simulink model "boostObserver_old"  (R2020a)
settings: Solver=VariableStepAuto  StartTime=0.0  StopTime=3.2  FixedStep=0.0005  MaxStep=9e-06  RelTol=1e-03  EnableMultiTasking=on
InitFcn:
  | kp=0.01;
  | ki=0.01;
  | 
  | k=2;
  | em=100000000;
  | GE=1/em;
  | GU=k*ki/GE;
  | GCE=k*kp/GU;
model workspace (MAT data in the model file):
  time = 0.8
values from neighbouring files (symbols this model uses):
  A1 = obj.boostConverter.A1    [BoostController.m]    (also in BoostConverter.m = [-obj.R/obj.L 0;0 -1/(obj.Ro*obj.C)]; BuckBoostConverter.m = [-obj.R/obj.L 0;0 -1/(obj.Ro*obj.C)]; obsmc.m = Asigma{1,1}; workspace_atual.mat = [-16.4  0; 0  -3.50877192982])
  A2 = obj.boostConverter.A2    [BoostController.m]    (also in BoostConverter.m = [-obj.R/obj.L -1/obj.L;1/obj.C -1/(obj.Ro*obj.C)]; BuckBoostConverter.m = [-obj.R/obj.L 1/obj.L;-1/obj.C -1/(obj.Ro*obj.C)]; obsmc.m = Asigma{1,2}; workspace_atual.mat = [-16.4  -200; 350.877192982  -3.50877192982])
  AlarmDeadTime = 0.50    (= 0.5)    [BoostFaultSimulation.m]    (also in workspace_atual.mat; workspace_certo.mat)
  B1 = obj.boostConverter.B1    [BoostController.m]    (also in BoostConverter.m = [1/obj.L;0]; BuckBoostConverter.m = [1/obj.L;0]; obsmc.m = Bsigma{1,1}; workspace_atual.mat = [200 0])
  boost_parameters = [obj.Ro,obj.R,obj.L,obj.C,obj.u]'    [BoostConverter.m]    (also in BuckBoostConverter.m; boostResults2Latex.m = boost.parameters(); workspace_atual.mat = [100 0.082 0.005 0.00285 190]; workspace_certo.mat = [100 0.082 0.005 0.00285 190])
  C = 1e-3    (= 0.001)    [boostResults2Latex.m]
  CiL = [0 1]    [workspace_atual.mat]    (also in workspace_certo.mat)
  Cmatrix = [1  0; 0  1]    [workspace_atual.mat]    (also in workspace_certo.mat)
  CVc = [1 0]    [workspace_atual.mat]    (also in workspace_certo.mat)
  D1 = [1  0; 0  1]    [workspace_atual.mat]    (also in workspace_certo.mat)
  FaultClass = 0    [BoostFaultSimulation.m]    (also in workspace_atual.mat = 1; workspace_certo.mat = 1)
  iLFaultSwitch = 0    [BoostFaultSimulation.m]    (also in workspace_atual.mat; workspace_certo.mat)
  iLFaultTime = 1.70    (= 1.7)    [BoostFaultSimulation.m]    (also in workspace_atual.mat; workspace_certo.mat)
  iLGainFaultFactor = 15    [BoostFaultSimulation.m]    (also in workspace_atual.mat; workspace_certo.mat)
  iLNoiseFaultSwitch = 0    [BoostFaultSimulation.m]    (also in workspace_atual.mat; workspace_certo.mat)
  iLNoiseTime = 1.70    (= 1.7)    [BoostFaultSimulation.m]    (also in workspace_atual.mat; workspace_certo.mat)
  Jth = 2000    [workspace_atual.mat]    (also in workspace_certo.mat)
  L = 1e-3    (= 0.001)    [boostResults2Latex.m]    (also in obsmc.m = sdpvar(3,1,'full'))
  LoadAddResistor = obj.LoadAddFactor*obj.Ro    [BoostFaultSimulation.m]    (also in workspace_atual.mat = 30; workspace_certo.mat = 30)
  LoadAddSignalSwitch = 1    [BoostFaultSimulation.m]    (also in workspace_atual.mat; workspace_certo.mat)
  LoadAddSwitch = 0    [BoostFaultSimulation.m]    (also in workspace_atual.mat; workspace_certo.mat)
  LoadAddTime = 0.90    (= 0.9)    [BoostFaultSimulation.m]    (also in workspace_atual.mat; workspace_certo.mat)
  LoadRemoveResistor = obj.Ro*(1-obj.LoadRemoveFactor)/(obj.LoadRemoveFactor)    [BoostFaultSimulation.m]    (also in workspace_atual.mat = 233.333333333; workspace_certo.mat = 233.333333333)
  LoadRemoveSignalSwitch = 1    [BoostFaultSimulation.m]    (also in workspace_atual.mat; workspace_certo.mat)
  LoadRemoveSwitch = 0    [BoostFaultSimulation.m]    (also in workspace_atual.mat; workspace_certo.mat)
  LoadRemoveTime = 0.90    (= 0.9)    [BoostFaultSimulation.m]    (also in workspace_atual.mat; workspace_certo.mat)
  LobsiL = [1737913.15707 66180.0912281]    [workspace_atual.mat]    (also in workspace_certo.mat)
  LobsVc = [61200 1]    [workspace_atual.mat]    (also in workspace_certo.mat)
  ObsEp = 70    [workspace_atual.mat]    (also in workspace_certo.mat)
  R = 0.1    [boostResults2Latex.m]    (also in workspace_atual.mat = 0.082; workspace_certo.mat = 0.082)
  ReconfigDelay = 0    [BoostFaultSimulation.m]    (also in workspace_atual.mat = 0.2; workspace_certo.mat = 0.2)
  ReconfigSwitch = 0    [BoostFaultSimulation.m]    (also in workspace_atual.mat; workspace_certo.mat)
  ReconfigTime = 1.707    [BoostFaultSimulation.m]    (also in workspace_atual.mat; workspace_certo.mat)
  rho = 5    [workspace_atual.mat]    (also in workspace_certo.mat)
  RMSfrequency = 47.61    [BoostFaultSimulation.m]    (also in workspace_atual.mat; workspace_certo.mat)
  Ro = 100    [BoostFaultSimulation.m]    (also in boostResults2Latex.m = 10; workspace_atual.mat; workspace_certo.mat)
  Smep = 80    [workspace_atual.mat]    (also in workspace_certo.mat)
  SourceAddSignalSwitch = 1    [BoostFaultSimulation.m]    (also in workspace_atual.mat; workspace_certo.mat)
  SourceAddSwitch = 0    [BoostFaultSimulation.m]    (also in workspace_atual.mat; workspace_certo.mat)
  SourceAddTime = 0.90    (= 0.9)    [BoostFaultSimulation.m]    (also in workspace_atual.mat; workspace_certo.mat)
  SourceAddVoltage = obj.SourceAddFactor*obj.u    [BoostFaultSimulation.m]    (also in workspace_atual.mat = 19; workspace_certo.mat = 19)
  SourceRemoveSignalSwitch = 1    [BoostFaultSimulation.m]    (also in workspace_atual.mat; workspace_certo.mat)
  SourceRemoveSwitch = 0    [BoostFaultSimulation.m]    (also in workspace_atual.mat; workspace_certo.mat)
  SourceRemoveTime = 0.90    (= 0.9)    [BoostFaultSimulation.m]    (also in workspace_atual.mat; workspace_certo.mat)
  SourceRemoveVoltage = obj.SourceRemoveFactor*obj.u    [BoostFaultSimulation.m]    (also in workspace_atual.mat = 19; workspace_certo.mat = 19)
  ueq = 0.5    [workspace_atual.mat]    (also in workspace_certo.mat)
  VcFaultSwitch = 0    [BoostFaultSimulation.m]    (also in workspace_atual.mat; workspace_certo.mat)
  VcFaultTime = 1.70    (= 1.7)    [BoostFaultSimulation.m]    (also in workspace_atual.mat; workspace_certo.mat)
  VcGainFaultFactor = 15    [BoostFaultSimulation.m]    (also in workspace_atual.mat; workspace_certo.mat)
  VcNoiseFaultSwitch = 0    [BoostFaultSimulation.m]    (also in workspace_atual.mat; workspace_certo.mat)
  VcNoiseTime = 1.70    (= 1.7)    [BoostFaultSimulation.m]    (also in workspace_atual.mat; workspace_certo.mat)
  ve = 380    [BoostFaultSimulation.m]    (also in boostResults2Latex.m = 100; workspace_atual.mat; workspace_certo.mat)
  x_e = [ie;ve]    [BoostConverter.m]    (also in BuckBoostConverter.m)
  xe = obj.boostConverter.equilibriumstate(ve)    [BoostController.m]    (also in workspace_atual.mat = [7.62509288104 380]; workspace_certo.mat = [7.62509288104 380])
undefined symbols (not defined in the file or in its folder): Atilde1, Atilde2, Ctilde1, Dtilde1, Dtilde2, F, G, MAXnet, MINnet
libraries: neural x74, powerlib x70, dspstat3 x16, simulink x9, powerlib_meascontrol x7, dspmtrx3 x7, dspmathops x3
(part 2 of 7)

== system boostObserver_old/Subsystem/Fault Identification Neural Netowrk ==
  netInputs : Inport
  Constant : Constant  Commented=on  Value=MAXnet
  Constant1 : Constant  Commented=on  Value=[0;0;0]
  Constant4 : Constant  Commented=on  Value=MINnet
  Demux : Demux  Commented=on  Outputs=3
  Demux1 : Demux  Commented=on  Outputs=3
  Demux2 : Demux  Commented=on  Outputs=3
  Maximum : dspstat3/Maximum  operation=maximum  fcn=Value and Index  indexBase=One  operateOver=Each column  Dimension=1  InputProcessing=Columns as channels (frame based)  reset=None  roiEnable=off  roiType=Rectangles  roiPortion=Entire ROI  roiOutput=Individual statistics for each ROI  roiFlag=off  roundingMode=Floor  overflowMode=off  accumDataTypeStr=Inherit: Same as product output  accumLastDataTypeStr=Inherit: Same as product output
  Median Filter : dspstat3/Median Filter  Commented=on  WindowLength=1  SimulateUsing=Code generation
      settings: SourceProductBaseCode=DS
  Mux : Mux  Commented=on  Inputs=3
  Pattern Recognition Neural Network1 : Subsystem
      mask help: Pattern Recognition Neural Network
      mask Display: e = 0.06;c1 = [120 150 230]/255;c2 = ([120 150 230]+0)/383;c3 = ([120 150 230]+128)/383;patch([0 1 1 0],[0 0 1 1],c1);patch([0 1 1 1-e 1-e 0+e],[0 0 1 1-e 0+e 0+e],c2);patch([0 0 1 1-e 0+e 0+e],[0 1 1 1-e 1-e 0+e],c3);plot([0 1 1 0 0],[0 0 1 1 0]);fprintf('NNET');port_label('input',1,' Input');port_label('output',1,'Output ');
  Scope : Scope
  Scope1 : Scope
  Subsystem : Subsystem  Commented=on
  Subsystem1 : Subsystem  Commented=on
  Subsystem2 : Subsystem  Commented=on
  Terminator : Terminator
  netOutputs : Outport
  wires:
  Maximum/1 -> Terminator/1
  Maximum/2 -> Scope1/1, netOutputs/1, Scope/1
  Constant/1 -> Demux/1
  Demux2/1 -> Subsystem/1(input)
  Demux1/1 -> Subsystem/2(min)
  Demux/1 -> Subsystem/3(max)
  Demux1/2 -> Subsystem1/2(min)
  Demux/2 -> Subsystem1/3(max)
  Demux2/2 -> Subsystem1/1(input)
  Demux/3 -> Subsystem2/3(max)
  Demux1/3 -> Subsystem2/2(min)
  Demux2/3 -> Subsystem2/1(input)
  Subsystem/1(Out1) -> Mux/1
  Subsystem1/1(Out1) -> Mux/2
  Subsystem2/1(Out1) -> Mux/3
  Constant4/1 -> Demux1/1
  netInputs/1 -> Pattern Recognition Neural Network1/1(Input)
  Pattern Recognition Neural Network1/1(Output) -> Maximum/1

== system boostObserver_old/Subsystem/If Action Subsystem ==
  In1 : Inport
  Action Port : ActionPort  ActionPortLabel=case [ 1 6 ]:
  Out1 : Outport
  wires:
  In1/1 -> Out1/1

== system boostObserver_old/Subsystem/If Action Subsystem1 ==
  In1 : Inport
  Action Port : ActionPort  ActionPortLabel=default:
  Out1 : Outport
  wires:
  In1/1 -> Out1/1

== system boostObserver_old/Subsystem/If Action Subsystem2 ==
  y : Inport
  Action Port : ActionPort  ActionPortLabel=case [ 4 5 ]:
  x_hat : Outport
  wires:
  y/1 -> x_hat/1

== system boostObserver_old/Subsystem/If Action Subsystem4 ==
  y : Inport
  Action Port : ActionPort  ActionPortLabel=case [ 2 3 ]:
  x_hat : Outport
  wires:
  y/1 -> x_hat/1

== system boostObserver_old/Subsystem/Residual Generator2 ==
  e_y : Inport
  Matrix Square1 : dspmtrx3/Matrix Square  OutMin=[]  OutMax=[]
      settings: SourceProductBaseCode=DS
  Moving RMS : dspstat3/Moving RMS  Method=Sliding window  ForgettingFactorPort=off  SpecifyWindowLength=on  WindowLength=RMSfrequency/10  ForgettingFactor=0.9  SimulateUsing=Code generation
      settings: SourceProductBaseCode=DS
  Sqrt2 : Sqrt  SaturateOnIntegerOverflow=on
  RMS : Outport
  wires:
  Matrix Square1/1 -> Sqrt2/1
  e_y/1 -> Matrix Square1/1
  Sqrt2/1 -> Moving RMS/1
  Moving RMS/1 -> RMS/1

== system boostObserver_old/Subsystem/Sliding Mode Observer 5 ==
  ey : Inport
  v : Inport  Port=2
  sigma : Inport  Port=3
  C : Constant  Value=Ctilde1
  ObserverDynamics : Subsystem
  Product : Product  Multiplication=Matrix(*)
  ey_out : Outport
  y_e_tilde_hat : Outport  Port=2
  wires:
  Product/1 -> y_e_tilde_hat/1
  C/1 -> Product/1
  ObserverDynamics/1(e_tilde_hat) -> Product/2
  sigma/1 -> ObserverDynamics/3(sigma)
  ey/1 -> ey_out/1, ObserverDynamics/1(ey)
  v/1 -> ObserverDynamics/2(v)

== system boostObserver_old/Subsystem/Subsystem ==
  y : Inport
  C : Inport  Port=2
  y_hat : Inport  Port=3
  "    1" : Constant  Value=ObsEp
  Product : Product  Multiplication=Matrix(*)
  SlidingSurface : Subsystem
  Subtract : Sum  Inputs=+-
  error : Outport
  wires:
  Subtract/1 -> SlidingSurface/1(S)  "y-y_hat"
  Product/1 -> Subtract/1
  "    1"/1 -> SlidingSurface/2(ep)
  SlidingSurface/1(d) -> error/1
  y_hat/1 -> Subtract/2
  C/1 -> Product/1
  y/1 -> Product/2

== system boostObserver_old/Subsystem/Subsystem1 ==
  y : Inport
  C : Inport  Port=2
  y_hat : Inport  Port=3
  "    1" : Constant  Value=ObsEp
  Product : Product  Multiplication=Matrix(*)
  SlidingSurface : Subsystem
  Subtract : Sum  Inputs=+-
  error : Outport
  wires:
  Subtract/1 -> SlidingSurface/1(S)  "y-y_hat"
  Product/1 -> Subtract/1
  "    1"/1 -> SlidingSurface/2(ep)
  SlidingSurface/1(d) -> error/1
  y_hat/1 -> Subtract/2
  C/1 -> Product/1
  y/1 -> Product/2

== system boostObserver_old/Subsystem/Subsystem2 ==
  x : Inport
  xe : Inport  Port=2
  y_fault : Inport  Port=3
  Constant : Constant  Value=D1
  Matrix Multiply : Product  Multiplication=Matrix(*)
  Sum : Sum  Inputs=|++
  Sum1 : Sum  Inputs=|-+
  y_e : Gain  Gain=Cmatrix  Multiplication=Matrix(K*u)
  f_s : Outport
  wires:
  Matrix Multiply/1 -> f_s/1
  Constant/1 -> Matrix Multiply/1  "D^- = D"
  x/1 -> Sum/1
  xe/1 -> Sum/2
  Sum/1 -> y_e/1
  y_e/1 -> Sum1/2
  Sum1/1 -> Matrix Multiply/2
  y_fault/1 -> Sum1/1

== system boostObserver_old/Subsystem/Subsystem9 ==
  x : Inport
  Demux : Demux  Outputs=2
  Residual Generator2 : Subsystem
  VcRMS : Outport
  wires:
  x/1 -> Demux/1
  Demux/2 -> Residual Generator2/1(e_y)
  Residual Generator2/1(RMS) -> VcRMS/1

== system boostObserver_old/Subsystem/Vc OBserver ==
  ObserverError : Inport
  C : Inport  Port=2
  sigma : Inport  Port=3
  Constant : Constant  Value=LobsVc
  Product2 : Product  Multiplication=Matrix(*)
  calc_x_hat : Subsystem
  x_hat : Outport
  y_hat : Outport  Port=2
  wires:
  sigma/1 -> calc_x_hat/1(sigma)
  calc_x_hat/1(x_hat) -> Product2/2, x_hat/1
  Product2/1 -> y_hat/1
  C/1 -> Product2/1
  ObserverError/1 -> calc_x_hat/2(rsign)
  Constant/1 -> calc_x_hat/3(Lobs)

== system boostObserver_old/Subsystem/iL Observer ==
  C : Inport
  ObserverError : Inport  Port=2
  sigma : Inport  Port=3
  Constant8 : Constant  Value=LobsiL
  Product2 : Product  Multiplication=Matrix(*)
  calc_x_hat : Subsystem
  x_hat : Outport
  y_hat : Outport  Port=2
  wires:
  sigma/1 -> calc_x_hat/1(sigma)
  calc_x_hat/1(x_hat) -> Product2/2, x_hat/1
  Product2/1 -> y_hat/1
  C/1 -> Product2/1
  ObserverError/1 -> calc_x_hat/2(rsign)
  Constant8/1 -> calc_x_hat/3(Lobs)

== system boostObserver_old/Subsystem3/AntiFalseAlarm ==
  PRNN : Inport
  Alarm : Inport  Port=2
  Constant7 : Constant
  FaultDetecition1 : Switch  Criteria=u2 > Threshold
  Product1 : Product
  Step1 : Step  Time=AlarmDeadTime  SampleTime=0
  FaultClass : Outport
  AlarmOut : Outport  Port=2
  wires:
  PRNN/1 -> FaultDetecition1/1
  Constant7/1 -> FaultDetecition1/3
  Step1/1 -> Product1/1
  Alarm/1 -> Product1/2
  Product1/1 -> AlarmOut/1, FaultDetecition1/2
  FaultDetecition1/1 -> FaultClass/1

== system boostObserver_old/Subsystem3/Augmented Error Generator ==
  e : Inport
  Mux : Mux  Inputs=2
  z1 : Subsystem
  e_tilde : Outport
  wires:
  z1/1(z) -> Mux/2
  Mux/1 -> e_tilde/1
  e/1 -> Mux/1, z1/1(z_dot)

== system boostObserver_old/Subsystem3/Boost Converter ==
  note: Escolha do tipo de entrada
  note: Circuito do conversor
  sigma : Inport
  ConversorBoost : Subsystem
  Mux1 : Mux  Inputs=2
  Terminator : Terminator
  Terminator1 : Terminator
  TipoEntrada : Subsystem
  x : Outport
  wires:
  TipoEntrada/4("Rvariavel ") -> [Rinput]
  sigma/1 -> ConversorBoost/1(sigma)
  [Vinput1] -> ConversorBoost/2(Vinput1)
  [Vinput2] -> ConversorBoost/3(Vinput2)
  [Rinput] -> ConversorBoost/5(Rinput)
  TipoEntrada/5("Rparallelvariavel ") -> [Rparallelinput]
  [Rparallelinput] -> ConversorBoost/6(Rparallelinput)
  [Vinput3] -> ConversorBoost/4(Vinput3)
  TipoEntrada/1(Vu) -> [Vinput1]
  TipoEntrada/2(VuAdd) -> [Vinput2]
  TipoEntrada/3(VuRemove) -> [Vinput3]
  ConversorBoost/1(iLoutput) -> Mux1/1
  ConversorBoost/2(Vcoutput) -> Mux1/2
  Mux1/1 -> x/1
  ConversorBoost/3(iro) -> Terminator/1
  ConversorBoost/4(Vu) -> Terminator1/1

== system boostObserver_old/Subsystem3/Controlador1 ==
  note: Sinal de controle
  note: Superfície
  note: Ponto de equilíbrio
  ve : Inport
  x : Inport  Port=2
  "    " : Constant  Value=ueq
  "    2" : Constant  Value=Smep
  Constant6 : Constant  Value=boost_parameters
  Demux1 : Demux  Outputs=2
  Demux2 : Demux  Outputs=2
  Gain : Gain  Gain=0.8
  Gain1 : Gain  Gain=8
  Gain3 : Gain  Gain=2.3
  Integrator1 : Integrator
  PWM : powerlib_meascontrol/Pulse & Signal Generators/PWM Generator (DC-DC)  Fsw=7000  Ts=0
  SlidingSurface : Subsystem
  Sum : Sum  Inputs=|++
  Sum4 : Sum  Inputs=++|
  Sum5 : Sum  Inputs=-+|
  Sum6 : Sum  Inputs=-+|
  Sum9 : Sum  Inputs=|++
  xe : MATLAB Function  TreatAsAtomicUnit=on
  sigma : Outport
  i_e : Outport  Port=2
  x_e : Outport  Port=3
  wires:
  Demux1/1 -> Sum6/2  "IL"
  PWM/1 -> sigma/1
  ve/1 -> xe/2(ve)
  Demux2/2 -> Sum5/1  "Vo1"
  "    "/1 -> Sum9/2
  Sum6/1 -> Gain1/1
  Sum5/1 -> Gain3/1, Gain/1
  Sum9/1 -> PWM/1
  Demux1/2 -> Sum5/2  "Vo1"
  Demux2/1 -> Sum6/1
  xe/2(i_e) -> i_e/1
  x/1 -> Demux2/1
  Constant6/1 -> xe/1(boost_parameters)
  Gain1/1 -> Sum4/2
  xe/1(x_e) -> Demux1/1, x_e/1
  Gain/1 -> Sum/1
  Gain3/1 -> Integrator1/1
  Sum/1 -> Sum4/1
  SlidingSurface/1(d) -> Sum9/1
  "    2"/1 -> SlidingSurface/2(ep)
  Sum4/1 -> SlidingSurface/1(S)
  Integrator1/1 -> Sum/2

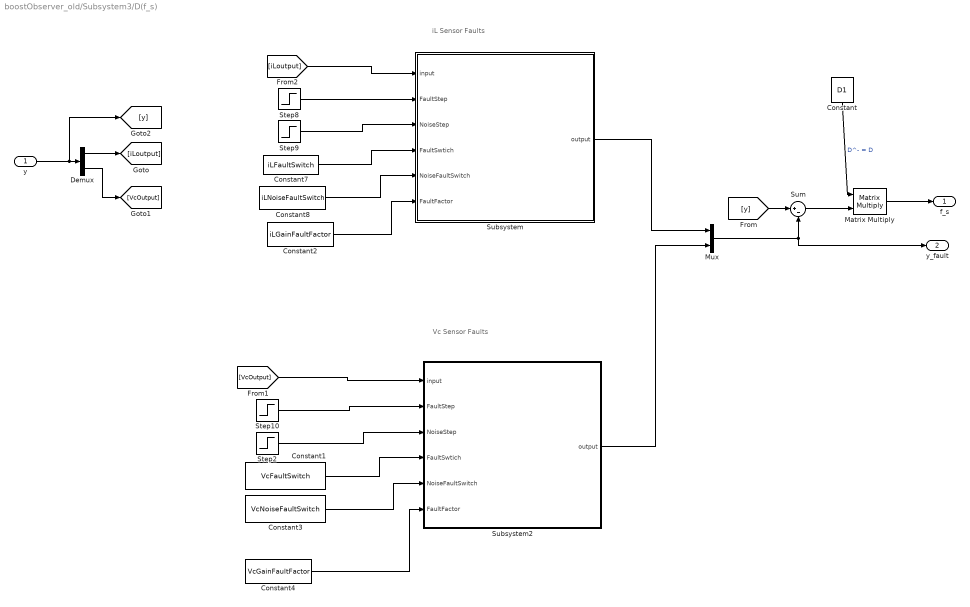
== system boostObserver_old/Subsystem3/D(f_s) ==
  note: iL Sensor Faults
  note: Vc Sensor Faults
  y : Inport
  Constant : Constant  Value=D1
  Constant1 : Constant  Value=VcFaultSwitch
  Constant2 : Constant  Value=iLGainFaultFactor
  Constant3 : Constant  Value=VcNoiseFaultSwitch
  Constant4 : Constant  Value=VcGainFaultFactor
  Constant7 : Constant  Value=iLFaultSwitch
  Constant8 : Constant  Value=iLNoiseFaultSwitch
  Demux : Demux  Outputs=2
  Matrix Multiply : Product  Multiplication=Matrix(*)
  Mux : Mux  Inputs=2
  Step10 : Step  Time=VcFaultTime  SampleTime=0
  Step2 : Step  Time=VcNoiseTime  SampleTime=0
  Step8 : Step  Time=iLFaultTime  SampleTime=0
  Step9 : Step  Time=iLNoiseTime  SampleTime=0
  Subsystem : Subsystem
  Subsystem2 : Subsystem
  Sum : Sum  Inputs=|+-
  f_s : Outport
  y_fault : Outport  Port=2
  wires:
  [iLoutput] -> Subsystem/1(input)
  Constant7/1 -> Subsystem/4(FaultSwtich)
  Constant8/1 -> Subsystem/5(NoiseFaultSwitch)
  Step8/1 -> Subsystem/2(FaultStep)
  Step9/1 -> Subsystem/3(NoiseStep)
  Constant1/1 -> Subsystem2/4(FaultSwtich)
  Constant3/1 -> Subsystem2/5(NoiseFaultSwitch)
  Step10/1 -> Subsystem2/2(FaultStep)
  Step2/1 -> Subsystem2/3(NoiseStep)
  Constant2/1 -> Subsystem/6(FaultFactor)
  Constant4/1 -> Subsystem2/6(FaultFactor)
  [VcOutput] -> Subsystem2/1(input)
  Demux/1 -> [iLoutput]
  Demux/2 -> [VcOutput]
  y/1 -> [y], Demux/1
  Subsystem/1(output) -> Mux/1
  Subsystem2/1(output) -> Mux/2
  Mux/1 -> Sum/2, y_fault/1
  [y] -> Sum/1
  Constant/1 -> Matrix Multiply/1  "D^- = D"
  Sum/1 -> Matrix Multiply/2
  Matrix Multiply/1 -> f_s/1

== system boostObserver_old/Subsystem3/ErrorGenerator ==
  y_e_tilde : Inport
  y_e_tilde_hat : Inport  Port=2
  AND : Logic  IconShape=distinctive  AllPortsSameDT=off  OutDataTypeStr=boolean
  Compare To Zero : simulink/Logic and Bit Operations/Compare To Zero  relop=~=  OutDataTypeStr=boolean
  Constant1 : Constant  Value=[0;0]
  Demux : Demux  Outputs=2
  If : If  IfExpression=u1 ~= 0
  If Action Subsystem : Subsystem  TreatAsAtomicUnit=on
  If Action Subsystem1 : Subsystem  TreatAsAtomicUnit=on
  Merge : Merge  InitialOutput=[0;0]
  Sum : Sum  Inputs=|+-
  e_y : Outport
  v : Outport  Port=2
  wires:
  y_e_tilde/1 -> Sum/1
  y_e_tilde_hat/1 -> Sum/2
  Sum/1 -> Compare To Zero/1, e_y/1, [e_y]
  If/1 -> If Action Subsystem/Action
  If/2 -> If Action Subsystem1/Action
  [e_y] -> If Action Subsystem/1(e_y)
  Constant1/1 -> If Action Subsystem1/1(e_y)
  If Action Subsystem/1(v) -> Merge/1
  If Action Subsystem1/1(v) -> Merge/2
  Demux/1 -> AND/1
  Demux/2 -> AND/2
  AND/1 -> If/1
  Merge/1 -> v/1
  Compare To Zero/1 -> Demux/1

== system boostObserver_old/Subsystem3/Fault Identification Neural Netowrk ==
  netInputs : Inport
  Maximum : dspstat3/Maximum  operation=maximum  fcn=Value and Index  indexBase=One  operateOver=Each column  Dimension=1  InputProcessing=Columns as channels (frame based)  reset=None  roiEnable=off  roiType=Rectangles  roiPortion=Entire ROI  roiOutput=Individual statistics for each ROI  roiFlag=off  roundingMode=Floor  overflowMode=off  accumDataTypeStr=Inherit: Same as product output  accumLastDataTypeStr=Inherit: Same as product output
  Median Filter : dspstat3/Median Filter  WindowLength=500  SimulateUsing=Code generation
      settings: SourceProductBaseCode=DS
  Pattern Recognition Neural Network : Subsystem  Commented=on
      mask help: Pattern Recognition Neural Network
      mask Display: e = 0.06;c1 = [120 150 230]/255;c2 = ([120 150 230]+0)/383;c3 = ([120 150 230]+128)/383;patch([0 1 1 0],[0 0 1 1],c1);patch([0 1 1 1-e 1-e 0+e],[0 0 1 1-e 0+e 0+e],c2);patch([0 0 1 1-e 0+e 0+e],[0 1 1 1-e 1-e 0+e],c3);plot([0 1 1 0 0],[0 0 1 1 0]);fprintf('NNET');port_label('input',1,' Input');port_label('output',1,'Output ');
  Pattern Recognition Neural Network Reconfig Big Data : Subsystem  Commented=on
      mask help: Pattern Recognition Neural Network
      mask Display: e = 0.06;c1 = [120 150 230]/255;c2 = ([120 150 230]+0)/383;c3 = ([120 150 230]+128)/383;patch([0 1 1 0],[0 0 1 1],c1);patch([0 1 1 1-e 1-e 0+e],[0 0 1 1-e 0+e 0+e],c2);patch([0 0 1 1-e 0+e 0+e],[0 1 1 1-e 1-e 0+e],c3);plot([0 1 1 0 0],[0 0 1 1 0]);fprintf('NNET');port_label('input',1,' Input');port_label('output',1,'Output ');
  Terminator : Terminator
  netOutputs : Outport
  wires:
  netInputs/1 -> Pattern Recognition Neural Network/1(Input)
  Maximum/1 -> Terminator/1
  Pattern Recognition Neural Network/1(Output) -> Maximum/1
  Maximum/2 -> Median Filter/1
  Median Filter/1 -> netOutputs/1

== system boostObserver_old/Subsystem3/If Action Subsystem ==
  In1 : Inport
  Action Port : ActionPort
  Constant : Constant  Value=0
  Out1 : Outport
  RESET : Outport  Port=2
  wires:
  In1/1 -> Out1/1
  Constant/1 -> RESET/1

== system boostObserver_old/Subsystem3/If Action Subsystem1 ==
  y : Inport
  clock : Inport  Port=2
  Action Port : ActionPort
  Cast To Double : DataTypeConversion  OutDataTypeStr=double
  Constant1 : Constant  Value=ReconfigDelay
  GetInitialTime : Subsystem
  GreaterThan : RelationalOperator  Operator=<=  OutDataTypeStr=boolean  RndMeth=Simplest
  Scope : Scope
  Scope1 : Scope
  Sum : Sum  Inputs=|++
  x_hat : Outport
  RESET : Outport  Port=2
  wires:
  Constant1/1 -> Sum/1
  [InitialTime] -> Sum/2
  Sum/1 -> Scope1/1, GreaterThan/2
  clock/1 -> GreaterThan/1, GetInitialTime/1(Clock)
  GetInitialTime/1(InitialTime) -> [InitialTime]
  y/1 -> x_hat/1
  GreaterThan/1 -> Scope/1, Cast To Double/1
  Cast To Double/1 -> RESET/1

== system boostObserver_old/Subsystem3/If Action Subsystem3 ==
  In1 : Inport
  Action Port : ActionPort
  Constant : Constant  Value=0
  Out1 : Outport
  RESET : Outport  Port=2
  wires:
  In1/1 -> Out1/1
  Constant/1 -> RESET/1

== system boostObserver_old/Subsystem3/If Action Subsystem4 ==
  y : Inport
  clock : Inport  Port=2
  Action Port : ActionPort
  Cast To Double : DataTypeConversion  OutDataTypeStr=double
  Constant1 : Constant  Value=ReconfigDelay
  GetInitialTime : Subsystem
  GreaterThan : RelationalOperator  Operator=<=  OutDataTypeStr=boolean  RndMeth=Simplest
  Sum : Sum  Inputs=|++
  x_hat : Outport
  RESET : Outport  Port=2
  wires:
  Constant1/1 -> Sum/1
  [InitialTime] -> Sum/2
  Sum/1 -> GreaterThan/2
  clock/1 -> GreaterThan/1, GetInitialTime/1(Clock)
  GetInitialTime/1(InitialTime) -> [InitialTime]
  y/1 -> x_hat/1
  GreaterThan/1 -> Cast To Double/1
  Cast To Double/1 -> RESET/1

== system boostObserver_old/Subsystem3/Residual Generator ==
  e_y : Inport
  Residual Generator1 : Subsystem
  RMS : Outport
  wires:
  e_y/1 -> Residual Generator1/1(e_y)
  Residual Generator1/1(RMS) -> RMS/1

== system boostObserver_old/Subsystem3/Sliding Mode Observer 5 ==
  ey : Inport
  v : Inport  Port=2
  sigma : Inport  Port=3
  C : Constant  Value=Ctilde1
  ObserverDynamics : Subsystem
  Product : Product  Multiplication=Matrix(*)
  ey_out : Outport
  y_e_tilde_hat : Outport  Port=2
  wires:
  Product/1 -> y_e_tilde_hat/1
  C/1 -> Product/1
  ObserverDynamics/1(e_tilde_hat) -> Product/2
  sigma/1 -> ObserverDynamics/3(sigma)
  ey/1 -> ey_out/1, ObserverDynamics/1(ey)
  v/1 -> ObserverDynamics/2(v)

== system boostObserver_old/Subsystem3/Subsystem ==
  y : Inport
  C : Inport  Port=2
  RESET : Inport  Port=3
  y_hat : Inport  Port=4
  "    1" : Constant  Value=ObsEp
  Constant : Constant  Value=xe  VectorParams1D=off  SampleTime=-1
  Product : Product  Multiplication=Matrix(*)
  SlidingSurface : Subsystem
  Subtract : Sum  Inputs=+-
  Switch : Switch  Criteria=u2 > Threshold
  error : Outport
  wires:
  Subtract/1 -> SlidingSurface/1(S)  "y-y_hat"
  Product/1 -> Subtract/1
  "    1"/1 -> SlidingSurface/2(ep)
  SlidingSurface/1(d) -> error/1
  y_hat/1 -> Subtract/2
  C/1 -> Product/1
  RESET/1 -> Switch/2
  y/1 -> Switch/3
  Switch/1 -> Product/2
  Constant/1 -> Switch/1

== system boostObserver_old/Subsystem3/Subsystem1 ==
  y : Inport
  C : Inport  Port=2
  RESET : Inport  Port=3
  y_hat : Inport  Port=4
  "    1" : Constant  Value=ObsEp
  Constant : Constant  Value=xe  VectorParams1D=off  SampleTime=-1
  Product : Product  Multiplication=Matrix(*)
  SlidingSurface : Subsystem
  Subtract : Sum  Inputs=+-
  Switch : Switch  Criteria=u2 > Threshold
  error : Outport
  wires:
  Subtract/1 -> SlidingSurface/1(S)  "y-y_hat"
  Product/1 -> Subtract/1
  "    1"/1 -> SlidingSurface/2(ep)
  SlidingSurface/1(d) -> error/1
  y_hat/1 -> Subtract/2
  C/1 -> Product/1
  RESET/1 -> Switch/2
  Constant/1 -> Switch/1
  y/1 -> Switch/3
  Switch/1 -> Product/2

== system boostObserver_old/Subsystem3/Subsystem9 ==
  x : Inport
  Demux : Demux  Outputs=2
  Residual Generator1 : Subsystem
  Residual Generator2 : Subsystem
  iLRMS : Outport
  VcRMS : Outport  Port=2
  wires:
  x/1 -> Demux/1
  Demux/1 -> Residual Generator2/1(e_y)
  Residual Generator2/1(RMS) -> iLRMS/1
  Demux/2 -> Residual Generator1/1(e_y)
  Residual Generator1/1(RMS) -> VcRMS/1

== system boostObserver_old/Subsystem3/Vc OBserver ==
  ObserverError : Inport
  C : Inport  Port=2
  sigma : Inport  Port=3
  Constant : Constant  Value=LobsVc
  Product2 : Product  Multiplication=Matrix(*)
  calc_x_hat : Subsystem
  x_hat : Outport
  y_hat : Outport  Port=2
  wires:
  sigma/1 -> calc_x_hat/1(sigma)
  calc_x_hat/1(x_hat) -> Product2/2, x_hat/1
  Product2/1 -> y_hat/1
  C/1 -> Product2/1
  ObserverError/1 -> calc_x_hat/2(rsign)
  Constant/1 -> calc_x_hat/3(Lobs)

== system boostObserver_old/Subsystem3/iL Observer ==
  C : Inport
  ObserverError : Inport  Port=2
  sigma : Inport  Port=3
  Constant8 : Constant  Value=LobsiL
  Product2 : Product  Multiplication=Matrix(*)
  calc_x_hat : Subsystem
  x_hat : Outport
  y_hat : Outport  Port=2
  wires:
  sigma/1 -> calc_x_hat/1(sigma)
  calc_x_hat/1(x_hat) -> Product2/2, x_hat/1
  Product2/1 -> y_hat/1
  C/1 -> Product2/1
  ObserverError/1 -> calc_x_hat/2(rsign)
  Constant8/1 -> calc_x_hat/3(Lobs)

== system boostObserver_old/reset/AntiFalseAlarm ==
  PRNN : Inport
  Alarm : Inport  Port=2
  Constant7 : Constant
  FaultDetecition1 : Switch  Criteria=u2 > Threshold
  Product1 : Product
  Step1 : Step  Time=AlarmDeadTime  SampleTime=0
  FaultClass : Outport
  AlarmOut : Outport  Port=2
  wires:
  PRNN/1 -> FaultDetecition1/1
  Constant7/1 -> FaultDetecition1/3
  Step1/1 -> Product1/1
  Alarm/1 -> Product1/2
  Product1/1 -> AlarmOut/1, FaultDetecition1/2
  FaultDetecition1/1 -> FaultClass/1

== system boostObserver_old/reset/Augmented Error Generator ==
  e : Inport
  Mux : Mux  Inputs=2
  z1 : Subsystem
  e_tilde : Outport
  wires:
  z1/1(z) -> Mux/2
  Mux/1 -> e_tilde/1
  e/1 -> Mux/1, z1/1(z_dot)

== system boostObserver_old/reset/Boost Converter ==
  note: Escolha do tipo de entrada
  note: Circuito do conversor
  sigma : Inport
  ConversorBoost : Subsystem
  Mux1 : Mux  Inputs=2
  Terminator : Terminator
  Terminator1 : Terminator
  TipoEntrada : Subsystem
  x : Outport
  wires:
  TipoEntrada/4("Rvariavel ") -> [Rinput]
  sigma/1 -> ConversorBoost/1(sigma)
  [Vinput1] -> ConversorBoost/2(Vinput1)
  [Vinput2] -> ConversorBoost/3(Vinput2)
  [Rinput] -> ConversorBoost/5(Rinput)
  TipoEntrada/5("Rparallelvariavel ") -> [Rparallelinput]
  [Rparallelinput] -> ConversorBoost/6(Rparallelinput)
  [Vinput3] -> ConversorBoost/4(Vinput3)
  TipoEntrada/1(Vu) -> [Vinput1]
  TipoEntrada/2(VuAdd) -> [Vinput2]
  TipoEntrada/3(VuRemove) -> [Vinput3]
  ConversorBoost/1(iLoutput) -> Mux1/1
  ConversorBoost/2(Vcoutput) -> Mux1/2
  Mux1/1 -> x/1
  ConversorBoost/3(iro) -> Terminator/1
  ConversorBoost/4(Vu) -> Terminator1/1

== system boostObserver_old/reset/Controlador1 ==
  note: Sinal de controle
  note: Superfície
  note: Ponto de equilíbrio
  ve : Inport
  x : Inport  Port=2
  "    " : Constant  Value=ueq
  "    2" : Constant  Value=Smep
  Constant6 : Constant  Value=boost_parameters
  Demux1 : Demux  Outputs=2
  Demux2 : Demux  Outputs=2
  Gain : Gain  Gain=0.8
  Gain1 : Gain  Gain=8
  Gain3 : Gain  Gain=2.3
  Integrator1 : Integrator
  PWM : powerlib_meascontrol/Pulse & Signal Generators/PWM Generator (DC-DC)  Fsw=7000  Ts=0
  Scope : Scope
  SlidingSurface : Subsystem
  Sum : Sum  Inputs=|++
  Sum4 : Sum  Inputs=++|
  Sum5 : Sum  Inputs=-+|
  Sum6 : Sum  Inputs=-+|
  Sum9 : Sum  Inputs=|++
  xe : MATLAB Function  TreatAsAtomicUnit=on
  sigma : Outport
  i_e : Outport  Port=2
  x_e : Outport  Port=3
  wires:
  Demux1/1 -> Sum6/2  "IL"
  PWM/1 -> sigma/1
  ve/1 -> xe/2(ve)
  Demux2/2 -> Sum5/1  "Vo1"
  "    "/1 -> Sum9/2
  Sum5/1 -> Gain3/1, Gain/1
  Sum9/1 -> PWM/1
  Demux1/2 -> Sum5/2  "Vo1"
  Demux2/1 -> Sum6/1
  xe/2(i_e) -> i_e/1
  x/1 -> Demux2/1
  Constant6/1 -> xe/1(boost_parameters)
  Gain1/1 -> Sum4/2
  xe/1(x_e) -> Demux1/1, x_e/1
  Gain/1 -> Sum/1
  Sum/1 -> Sum4/1
  SlidingSurface/1(d) -> Scope/1, Sum9/1
  "    2"/1 -> SlidingSurface/2(ep)
  Sum6/1 -> Gain1/1
  Gain3/1 -> Integrator1/1
  Integrator1/1 -> Sum/2
  Sum4/1 -> SlidingSurface/1(S)

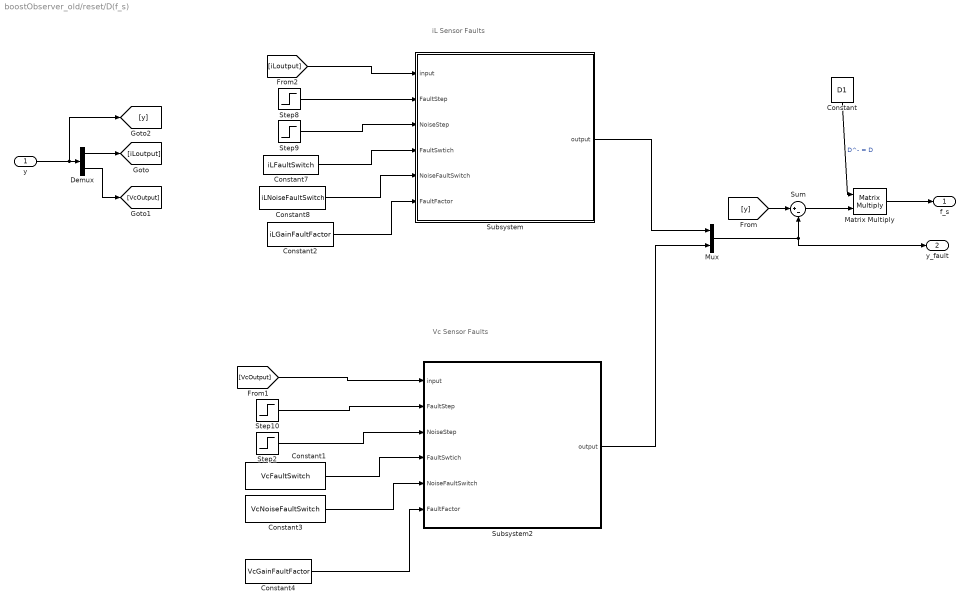
== system boostObserver_old/reset/D(f_s) ==
  note: iL Sensor Faults
  note: Vc Sensor Faults
  y : Inport
  Constant : Constant  Value=D1
  Constant1 : Constant  Value=VcFaultSwitch
  Constant2 : Constant  Value=iLGainFaultFactor
  Constant3 : Constant  Value=VcNoiseFaultSwitch
  Constant4 : Constant  Value=VcGainFaultFactor
  Constant7 : Constant  Value=iLFaultSwitch
  Constant8 : Constant  Value=iLNoiseFaultSwitch
  Demux : Demux  Outputs=2
  Matrix Multiply : Product  Multiplication=Matrix(*)
  Mux : Mux  Inputs=2
  Step10 : Step  Time=VcFaultTime  SampleTime=0
  Step2 : Step  Time=VcNoiseTime  SampleTime=0
  Step8 : Step  Time=iLFaultTime  SampleTime=0
  Step9 : Step  Time=iLNoiseTime  SampleTime=0
  Subsystem : Subsystem
  Subsystem2 : Subsystem
  Sum : Sum  Inputs=|+-
  f_s : Outport
  y_fault : Outport  Port=2
  wires:
  [iLoutput] -> Subsystem/1(input)
  Constant7/1 -> Subsystem/4(FaultSwtich)
  Constant8/1 -> Subsystem/5(NoiseFaultSwitch)
  Step8/1 -> Subsystem/2(FaultStep)
  Step9/1 -> Subsystem/3(NoiseStep)
  Constant1/1 -> Subsystem2/4(FaultSwtich)
  Constant3/1 -> Subsystem2/5(NoiseFaultSwitch)
  Step10/1 -> Subsystem2/2(FaultStep)
  Step2/1 -> Subsystem2/3(NoiseStep)
  Constant2/1 -> Subsystem/6(FaultFactor)
  Constant4/1 -> Subsystem2/6(FaultFactor)
  [VcOutput] -> Subsystem2/1(input)
  Demux/1 -> [iLoutput]
  Demux/2 -> [VcOutput]
  y/1 -> [y], Demux/1
  Subsystem/1(output) -> Mux/1
  Subsystem2/1(output) -> Mux/2
  Mux/1 -> Sum/2, y_fault/1
  [y] -> Sum/1
  Constant/1 -> Matrix Multiply/1  "D^- = D"
  Sum/1 -> Matrix Multiply/2
  Matrix Multiply/1 -> f_s/1

== system boostObserver_old/reset/ErrorGenerator ==
  y_e_tilde : Inport
  y_e_tilde_hat : Inport  Port=2
  AND : Logic  IconShape=distinctive  AllPortsSameDT=off  OutDataTypeStr=boolean
  Compare To Zero : simulink/Logic and Bit Operations/Compare To Zero  relop=~=  OutDataTypeStr=boolean
  Constant1 : Constant  Value=[0;0]
  Demux : Demux  Outputs=2
  If : If  IfExpression=u1 ~= 0
  If Action Subsystem : Subsystem  TreatAsAtomicUnit=on
  If Action Subsystem1 : Subsystem  TreatAsAtomicUnit=on
  Merge : Merge  InitialOutput=[0;0]
  Sum : Sum  Inputs=|+-
  e_y : Outport
  v : Outport  Port=2
  wires:
  y_e_tilde/1 -> Sum/1
  y_e_tilde_hat/1 -> Sum/2
  Sum/1 -> Compare To Zero/1, e_y/1, [e_y]
  If/1 -> If Action Subsystem/Action
  If/2 -> If Action Subsystem1/Action
  [e_y] -> If Action Subsystem/1(e_y)
  Constant1/1 -> If Action Subsystem1/1(e_y)
  If Action Subsystem/1(v) -> Merge/1
  If Action Subsystem1/1(v) -> Merge/2
  Demux/1 -> AND/1
  Demux/2 -> AND/2
  AND/1 -> If/1
  Merge/1 -> v/1
  Compare To Zero/1 -> Demux/1

== system boostObserver_old/reset/Fault Identification Neural Netowrk ==
  netInputs : Inport
  Maximum : dspstat3/Maximum  operation=maximum  fcn=Value and Index  indexBase=One  operateOver=Each column  Dimension=1  InputProcessing=Columns as channels (frame based)  reset=None  roiEnable=off  roiType=Rectangles  roiPortion=Entire ROI  roiOutput=Individual statistics for each ROI  roiFlag=off  roundingMode=Floor  overflowMode=off  accumDataTypeStr=Inherit: Same as product output  accumLastDataTypeStr=Inherit: Same as product output
  Median Filter : dspstat3/Median Filter  WindowLength=300  SimulateUsing=Code generation
      settings: SourceProductBaseCode=DS
  Pattern Recognition Neural Network2 : Subsystem  Commented=on
      mask help: Pattern Recognition Neural Network
      mask Display: e = 0.06;c1 = [120 150 230]/255;c2 = ([120 150 230]+0)/383;c3 = ([120 150 230]+128)/383;patch([0 1 1 0],[0 0 1 1],c1);patch([0 1 1 1-e 1-e 0+e],[0 0 1 1-e 0+e 0+e],c2);patch([0 0 1 1-e 0+e 0+e],[0 1 1 1-e 1-e 0+e],c3);plot([0 1 1 0 0],[0 0 1 1 0]);fprintf('NNET');port_label('input',1,' Input');port_label('output',1,'Output ');
  Pattern Recognition Neural Network3 : Subsystem
      mask help: Pattern Recognition Neural Network
      mask Display: e = 0.06;c1 = [120 150 230]/255;c2 = ([120 150 230]+0)/383;c3 = ([120 150 230]+128)/383;patch([0 1 1 0],[0 0 1 1],c1);patch([0 1 1 1-e 1-e 0+e],[0 0 1 1-e 0+e 0+e],c2);patch([0 0 1 1-e 0+e 0+e],[0 1 1 1-e 1-e 0+e],c3);plot([0 1 1 0 0],[0 0 1 1 0]);fprintf('NNET');port_label('input',1,' Input');port_label('output',1,'Output ');
  Terminator : Terminator
  netOutputs : Outport
  wires:
  Maximum/1 -> Terminator/1
  netInputs/1 -> Pattern Recognition Neural Network3/1(Input)
  Pattern Recognition Neural Network3/1(Output) -> Maximum/1
  Maximum/2 -> Median Filter/1
  Median Filter/1 -> netOutputs/1

== system boostObserver_old/reset/If Action Subsystem ==
  In1 : Inport
  Action Port : ActionPort  ActionPortLabel=case [ 1 6 ]:
  Constant : Constant  Value=0
  Out1 : Outport
  RESET : Outport  Port=2
  wires:
  In1/1 -> Out1/1
  Constant/1 -> RESET/1

== system boostObserver_old/reset/If Action Subsystem1 ==
  y : Inport
  clock : Inport  Port=2
  Action Port : ActionPort  ActionPortLabel=case [ 4 5 ]:
  Cast To Double : DataTypeConversion  OutDataTypeStr=double
  Constant1 : Constant  Value=ReconfigDelay
  GetInitialTime : Subsystem
  GreaterThan : RelationalOperator  Operator=<  OutDataTypeStr=boolean  RndMeth=Simplest
  Sum : Sum  Inputs=|++
  x_hat : Outport
  RESET : Outport  Port=2
  wires:
  Constant1/1 -> Sum/1
  [InitialTime] -> Sum/2
  Sum/1 -> GreaterThan/2
  clock/1 -> GreaterThan/1, GetInitialTime/1(Clock)
  GetInitialTime/1(InitialTime) -> [InitialTime]
  y/1 -> x_hat/1
  GreaterThan/1 -> Cast To Double/1
  Cast To Double/1 -> RESET/1

== system boostObserver_old/reset/If Action Subsystem3 ==
  In1 : Inport
  Action Port : ActionPort  ActionPortLabel=default:
  Constant : Constant  Value=0
  Out1 : Outport
  RESET : Outport  Port=2
  wires:
  In1/1 -> Out1/1
  Constant/1 -> RESET/1

== system boostObserver_old/reset/If Action Subsystem4 ==
  y : Inport
  clock : Inport  Port=2
  Action Port : ActionPort  ActionPortLabel=case [ 2 3 ]:
  Cast To Double : DataTypeConversion  OutDataTypeStr=double
  Constant1 : Constant  Value=ReconfigDelay
  GetInitialTime : Subsystem
  GreaterThan : RelationalOperator  Operator=<  OutDataTypeStr=boolean  RndMeth=Simplest
  Sum : Sum  Inputs=|++
  x_hat : Outport
  RESET : Outport  Port=2
  wires:
  Constant1/1 -> Sum/1
  [InitialTime] -> Sum/2
  Sum/1 -> GreaterThan/2
  clock/1 -> GreaterThan/1, GetInitialTime/1(Clock)
  GetInitialTime/1(InitialTime) -> [InitialTime]
  y/1 -> x_hat/1
  GreaterThan/1 -> Cast To Double/1
  Cast To Double/1 -> RESET/1

== system boostObserver_old/reset/Residual Generator2 ==
  e_y : Inport
  Matrix Square1 : dspmtrx3/Matrix Square  OutMin=[]  OutMax=[]
      settings: SourceProductBaseCode=DS
  Moving RMS : dspstat3/Moving RMS  Method=Sliding window  ForgettingFactorPort=off  SpecifyWindowLength=on  WindowLength=RMSfrequency/10  ForgettingFactor=0.9  SimulateUsing=Code generation
      settings: SourceProductBaseCode=DS
  Sqrt2 : Sqrt  SaturateOnIntegerOverflow=on
  RMS : Outport
  wires:
  Matrix Square1/1 -> Sqrt2/1
  Sqrt2/1 -> Moving RMS/1
  e_y/1 -> Matrix Square1/1
  Moving RMS/1 -> RMS/1

== system boostObserver_old/reset/Residual Generator3 ==
  e_y : Inport
  Matrix Square1 : dspmtrx3/Matrix Square  OutMin=[]  OutMax=[]
      settings: SourceProductBaseCode=DS
  Moving RMS : dspstat3/Moving RMS  Method=Sliding window  ForgettingFactorPort=off  SpecifyWindowLength=on  WindowLength=RMSfrequency  ForgettingFactor=0.9  SimulateUsing=Code generation
      settings: SourceProductBaseCode=DS
  Sqrt2 : Sqrt  SaturateOnIntegerOverflow=on
  RMS : Outport
  wires:
  Matrix Square1/1 -> Sqrt2/1
  Sqrt2/1 -> Moving RMS/1
  e_y/1 -> Matrix Square1/1
  Moving RMS/1 -> RMS/1

== system boostObserver_old/reset/Sliding Mode Observer 5 ==
  ey : Inport
  v : Inport  Port=2
  sigma : Inport  Port=3
  C : Constant  Value=Ctilde1
  ObserverDynamics : Subsystem
  Product : Product  Multiplication=Matrix(*)
  ey_out : Outport
  y_e_tilde_hat : Outport  Port=2
  wires:
  Product/1 -> y_e_tilde_hat/1
  C/1 -> Product/1
  ObserverDynamics/1(e_tilde_hat) -> Product/2
  sigma/1 -> ObserverDynamics/3(sigma)
  ey/1 -> ey_out/1, ObserverDynamics/1(ey)
  v/1 -> ObserverDynamics/2(v)

== system boostObserver_old/reset/Subsystem ==
  y : Inport
  C : Inport  Port=2
  RESET : Inport  Port=3
  y_hat : Inport  Port=4
  "    1" : Constant  Value=ObsEp
  Constant : Constant  Value=xe  VectorParams1D=off  SampleTime=-1
  Product : Product  Multiplication=Matrix(*)
  SlidingSurface : Subsystem
  Subtract : Sum  Inputs=+-
  Switch : Switch  Criteria=u2 > Threshold
  error : Outport
  wires:
  Subtract/1 -> SlidingSurface/1(S)  "y-y_hat"
  Product/1 -> Subtract/1
  "    1"/1 -> SlidingSurface/2(ep)
  SlidingSurface/1(d) -> error/1
  y_hat/1 -> Subtract/2
  C/1 -> Product/1
  RESET/1 -> Switch/2
  y/1 -> Switch/3
  Switch/1 -> Product/2
  Constant/1 -> Switch/1

== system boostObserver_old/reset/Subsystem1 ==
  y : Inport
  C : Inport  Port=2
  RESET : Inport  Port=3
  y_hat : Inport  Port=4
  "    1" : Constant  Value=ObsEp
  Constant : Constant  Value=xe  VectorParams1D=off  SampleTime=-1
  Product : Product  Multiplication=Matrix(*)
  SlidingSurface : Subsystem
  Subtract : Sum  Inputs=+-
  Switch : Switch  Criteria=u2 > Threshold
  error : Outport
  wires:
  Subtract/1 -> SlidingSurface/1(S)  "y-y_hat"
  Product/1 -> Subtract/1
  "    1"/1 -> SlidingSurface/2(ep)
  SlidingSurface/1(d) -> error/1
  y_hat/1 -> Subtract/2
  C/1 -> Product/1
  RESET/1 -> Switch/2
  Constant/1 -> Switch/1
  y/1 -> Switch/3
  Switch/1 -> Product/2

== system boostObserver_old/reset/Subsystem9 ==
  x : Inport
  Demux : Demux  Outputs=2
  Residual Generator1 : Subsystem
  Residual Generator2 : Subsystem
  Scope : Scope
  iLRMS : Outport
  VcRMS : Outport  Port=2
  wires:
  x/1 -> Demux/1
  Demux/2 -> Residual Generator1/1(e_y)
  Residual Generator1/1(RMS) -> VcRMS/1
  Demux/1 -> Residual Generator2/1(e_y)
  Residual Generator2/1(RMS) -> Scope/1, iLRMS/1

== system boostObserver_old/reset/Vc OBserver ==
  ObserverError : Inport
  C : Inport  Port=2
  sigma : Inport  Port=3
  Constant : Constant  Value=LobsVc
  Product2 : Product  Multiplication=Matrix(*)
  calc_x_hat : Subsystem
  x_hat : Outport
  y_hat : Outport  Port=2
  wires:
  sigma/1 -> calc_x_hat/1(sigma)
  calc_x_hat/1(x_hat) -> Product2/2, x_hat/1
  Product2/1 -> y_hat/1
  C/1 -> Product2/1
  ObserverError/1 -> calc_x_hat/2(rsign)
  Constant/1 -> calc_x_hat/3(Lobs)

== system boostObserver_old/reset/iL Observer ==
  C : Inport
  ObserverError : Inport  Port=2
  sigma : Inport  Port=3
  Constant8 : Constant  Value=LobsiL
  Product2 : Product  Multiplication=Matrix(*)
  calc_x_hat : Subsystem
  x_hat : Outport
  y_hat : Outport  Port=2
  wires:
  sigma/1 -> calc_x_hat/1(sigma)
  calc_x_hat/1(x_hat) -> Product2/2, x_hat/1
  Product2/1 -> y_hat/1
  C/1 -> Product2/1
  ObserverError/1 -> calc_x_hat/2(rsign)
  Constant8/1 -> calc_x_hat/3(Lobs)

== system boostObserver_old/Subsystem/Augmented Error Generator/z1 ==
  z_dot : Inport
  Constant1 : Constant  Value=[0;0]  VectorParams1D=off
  Gain2 : Gain  Gain=Cmatrix  Multiplication=Matrix(K*u) (u vector)
  Integrator6 : Integrator  InitialConditionSource=external
  z : Outport
  wires:
  Gain2/1 -> Integrator6/1
  Integrator6/1 -> z/1
  z_dot/1 -> Gain2/1
  Constant1/1 -> Integrator6/2

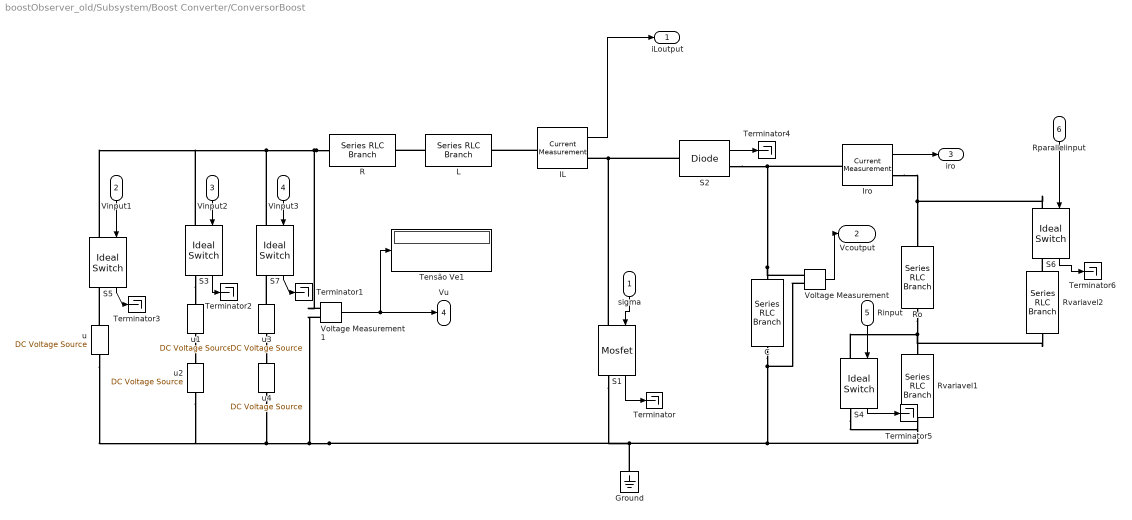
== system boostObserver_old/Subsystem/Boost Converter/ConversorBoost ==
  sigma : Inport
  Vinput1 : Inport  Port=2
  Vinput2 : Inport  Port=3
  Vinput3 : Inport  Port=4
  Rinput : Inport  Port=5
  Rparallelinput : Inport  Port=6
  C : powerlib/Elements/Series RLC Branch  LConnTagsString=__new0  RConnTagsString=__new0  BranchType=C  Resistance=1  Inductance=1e-3  SetiL0=off  InitialCurrent=0  Capacitance=C  Setx0=on  InitialVoltage=0  Measurements=None
  Ground : powerlib/Elements/Ground  LConnTagsString=a
  IL : powerlib/Measurements/Current Measurement  PhasorSimulation=off  OutputType=Complex  PSBequivalent=0
  Iro : powerlib/Measurements/Current Measurement  PhasorSimulation=off  OutputType=Complex  PSBequivalent=0
  L : powerlib/Elements/Series RLC Branch  LConnTagsString=__new0  RConnTagsString=__new0  BranchType=L  Resistance=1  Inductance=L  SetiL0=on  InitialCurrent=0  Capacitance=1e-6  Setx0=off  InitialVoltage=0  Measurements=None
  R : powerlib/Elements/Series RLC Branch  LConnTagsString=__new0  RConnTagsString=__new0  BranchType=R  Resistance=R  Inductance=1e-3  SetiL0=off  InitialCurrent=0  Capacitance=1e-6  Setx0=off  InitialVoltage=0  Measurements=None
  Ro : powerlib/Elements/Series RLC Branch  LConnTagsString=__new0  RConnTagsString=__new0  BranchType=R  Resistance=Ro  Inductance=1e-3  SetiL0=off  InitialCurrent=0  Capacitance=1e-6  Setx0=off  InitialVoltage=0  Measurements=None
  Rvariavel1 : powerlib/Elements/Series RLC Branch  LConnTagsString=__new0  RConnTagsString=__new0  BranchType=R  Resistance=LoadAddResistor  Inductance=1e-3  SetiL0=off  InitialCurrent=0  Capacitance=1e-6  Setx0=off  InitialVoltage=0  Measurements=None
  Rvariavel2 : powerlib/Elements/Series RLC Branch  LConnTagsString=__new0  RConnTagsString=__new0  BranchType=R  Resistance=LoadRemoveResistor  Inductance=1e-3  SetiL0=off  InitialCurrent=0  Capacitance=1e-6  Setx0=off  InitialVoltage=0  Measurements=None
  S1 : powerlib/Power Electronics/Mosfet  Ron=0.0000001  Lon=0  Rd=0.000000001  Vfd=0  IC=0  Rs=1e5  Cs=inf  Measurements=on
  S2 : powerlib/Power Electronics/Diode  Ron=0.000001  Lon=0  Vf=0  IC=0  UseSnubber=off  Rs=0  Cs=0  Measurements=on
  S{3..7} (5 alike) : powerlib/Power Electronics/Ideal Switch  Ron=0.0000001  Lon=0  IC=0  Rs=1e8  Cs=inf  Measurements=on
  Tensão Ve1 : Display
  Terminator{,1..6} (7 alike) : Terminator
  Voltage Measurement : powerlib/Measurements/Voltage Measurement  PhasorSimulation=off  OutputType=Complex  PSBequivalent=0
  Voltage Measurement1 : powerlib/Measurements/Voltage Measurement  PhasorSimulation=off  OutputType=Complex  PSBequivalent=0
  u : powerlib/Electrical Sources/DC Voltage Source  Amplitude=u  Measurements=None
  u1 : powerlib/Electrical Sources/DC Voltage Source  Amplitude=SourceAddVoltage  Measurements=None
  u2 : powerlib/Electrical Sources/DC Voltage Source  Amplitude=u  Measurements=None
  u3 : powerlib/Electrical Sources/DC Voltage Source  Amplitude=SourceRemoveVoltage  Measurements=None
  u4 : powerlib/Electrical Sources/DC Voltage Source  Amplitude=u  Measurements=None
  iLoutput : Outport
  Vcoutput : Outport  Port=2
  iro : Outport  Port=3
  Vu : Outport  Port=4
  wires:
  Rinput/1 -> S4/1
  IL/1 -> iLoutput/1
  sigma/1 -> S1/1
  Voltage Measurement/1 -> Vcoutput/1
  Iro/1 -> iro/1
  Voltage Measurement1/1 -> Vu/1, Tensão Ve1/1
  Vinput1/1 -> S5/1
  Vinput2/1 -> S3/1
  Rparallelinput/1 -> S6/1
  Vinput3/1 -> S7/1
  S1/1 -> Terminator/1
  S7/1 -> Terminator1/1
  S3/1 -> Terminator2/1
  S5/1 -> Terminator3/1
  S2/1 -> Terminator4/1
  S4/1 -> Terminator5/1
  S6/1 -> Terminator6/1
  connections:
  Ro/RConn1 -- Rvariavel2/LConn1 -- Rvariavel1/RConn1 -- S4/LConn1
  IL/LConn1 -- L/RConn1
  C/RConn1 -- S4/RConn1 -- Rvariavel1/LConn1 -- S1/RConn1 -- u2/LConn1 -- u/LConn1 -- u4/LConn1 -- Voltage Measurement1/LConn2 -- Ground/LConn1 -- Voltage Measurement/LConn2
  S2/LConn1 -- S1/LConn1 -- IL/RConn1
  R/LConn1 -- S3/LConn1 -- S5/LConn1 -- S7/LConn1 -- Voltage Measurement1/LConn1
  Iro/RConn1 -- S6/LConn1 -- Ro/LConn1
  L/LConn1 -- R/RConn1
  S2/RConn1 -- Iro/LConn1 -- Voltage Measurement/LConn1 -- C/LConn1
  u/RConn1 -- S5/RConn1
  Rvariavel2/RConn1 -- S6/RConn1
  S3/RConn1 -- u1/RConn1
  u1/LConn1 -- u2/RConn1
  u3/LConn1 -- S7/RConn1
  u3/RConn1 -- u4/RConn1

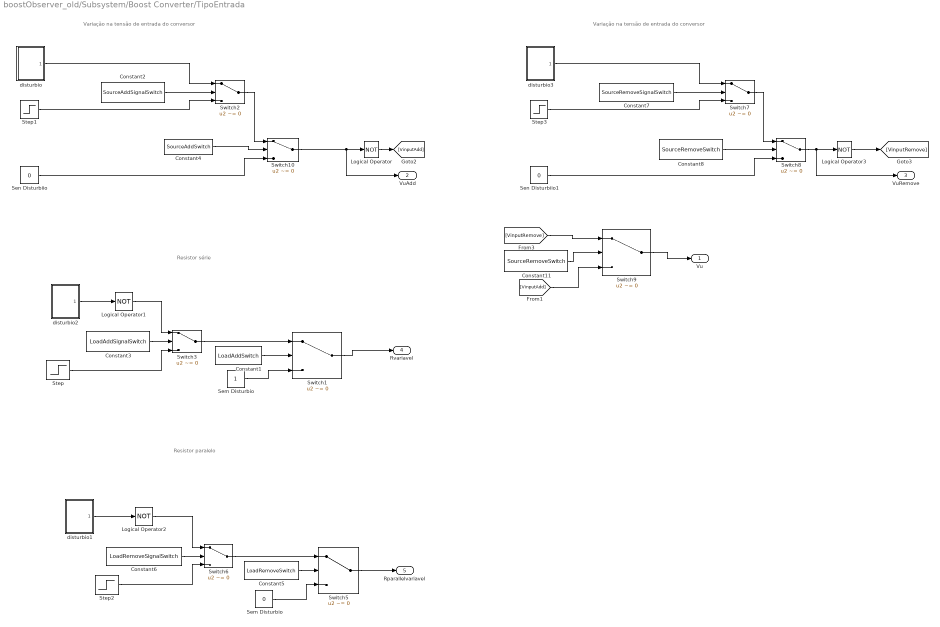
== system boostObserver_old/Subsystem/Boost Converter/TipoEntrada ==
  note: Variação na tensão de entrada do conversor
  note: Resistor série
  note: Resistor paralelo
  note: Variação na tensão de entrada do conversor
  Constant1 : Constant  Value=LoadAddSwitch
  Constant11 : Constant  Value=SourceRemoveSwitch
  Constant2 : Constant  Value=SourceAddSignalSwitch
  Constant3 : Constant  Value=LoadAddSignalSwitch
  Constant4 : Constant  Value=SourceAddSwitch
  Constant5 : Constant  Value=LoadRemoveSwitch
  Constant6 : Constant  Value=LoadRemoveSignalSwitch
  Constant7 : Constant  Value=SourceRemoveSignalSwitch
  Constant8 : Constant  Value=SourceRemoveSwitch
  Logical Operator{,1..3} (4 alike) : Logic  Operator=NOT  AllPortsSameDT=off  OutDataTypeStr=boolean
  Sem Disturbio : Constant
  "Sem Disturbio  " : Constant  Value=0
  Sen Disturbiio : Constant  Value=0
  Sen Disturbiio1 : Constant  Value=0
  Step : Step  Time=LoadAddTime  Before=1  After=0  SampleTime=0
  Step1 : Step  Time=SourceAddTime  SampleTime=0
  Step2 : Step  Time=LoadRemoveTime  SampleTime=0
  Step3 : Step  Time=SourceRemoveTime  SampleTime=0
  Switch{1..3,5..10} (9 alike) : Switch  Criteria=u2 ~= 0
  disturbio : Subsystem
  disturbio1 : Subsystem
  disturbio2 : Subsystem
  disturbio3 : Subsystem
  Vu : Outport
  VuAdd : Outport  Port=2
  VuRemove : Outport  Port=3
  "Rvariavel " : Outport  Port=4
  "Rparallelvariavel " : Outport  Port=5
  wires:
  Sen Disturbiio/1 -> Switch10/3
  Constant4/1 -> Switch10/2
  Constant1/1 -> Switch1/2
  Switch1/1 -> "Rvariavel "/1
  Constant2/1 -> Switch2/2
  Constant3/1 -> Switch3/2
  Switch2/1 -> Switch10/1
  disturbio2/1(disturbio) -> Logical Operator1/1
  Switch3/1 -> Switch1/1
  Sem Disturbio/1 -> Switch1/3
  Switch6/1 -> Switch5/1
  disturbio1/1(disturbio) -> Logical Operator2/1
  Constant6/1 -> Switch6/2
  "Sem Disturbio  "/1 -> Switch5/3
  Switch5/1 -> "Rparallelvariavel "/1
  Constant5/1 -> Switch5/2
  disturbio/1(disturbio) -> Switch2/1
  Step1/1 -> Switch2/3
  Logical Operator1/1 -> Switch3/1
  Step/1 -> Switch3/3
  Step2/1 -> Switch6/3
  Logical Operator2/1 -> Switch6/1
  disturbio3/1(disturbio) -> Switch7/1
  Constant8/1 -> Switch8/2
  Constant7/1 -> Switch7/2
  Switch8/1 -> VuRemove/1, Logical Operator3/1
  Sen Disturbiio1/1 -> Switch8/3
  Switch7/1 -> Switch8/1
  Step3/1 -> Switch7/3
  [VinputAdd] -> Switch9/3
  Constant11/1 -> Switch9/2
  Switch10/1 -> VuAdd/1, Logical Operator/1
  Switch9/1 -> Vu/1
  Logical Operator/1 -> [VinputAdd]
  Logical Operator3/1 -> [VinputRemove]
  [VinputRemove] -> Switch9/1

== system boostObserver_old/Subsystem/Controlador1/SlidingSurface ==
  S : Inport
  ep : Inport  Port=2
  Abs : Abs
  GreaterThan : RelationalOperator  Operator=>  OutDataTypeStr=boolean  RndMeth=Simplest
  If : If  IfExpression=u1 ~= 0
  If Action Subsystem : Subsystem  TreatAsAtomicUnit=on
  If Action Subsystem2 : Subsystem  TreatAsAtomicUnit=on
  Merge1 : Merge
  d : Outport
  wires:
  If Action Subsystem2/1(d) -> Merge1/2
  [S] -> If Action Subsystem/1(S), If Action Subsystem2/1(S)
  If/2 -> If Action Subsystem2/Action
  If/1 -> If Action Subsystem/Action
  [ep] -> If Action Subsystem2/2(ep)
  S/1 -> [S], Abs/1
  If Action Subsystem/1(d) -> Merge1/1
  Abs/1 -> GreaterThan/1
  GreaterThan/1 -> If/1
  Merge1/1 -> d/1
  ep/1 -> [ep], GreaterThan/2

== system boostObserver_old/Subsystem/D(f_s)/Subsystem ==
  input : Inport
  FaultStep : Inport  Port=2
  NoiseStep : Inport  Port=3
  FaultSwtich : Inport  Port=4
  NoiseFaultSwitch : Inport  Port=5
  FaultFactor : Inport  Port=6
  Constant11 : Constant  Value=0
  Constant9 : Constant  Value=0
  Product : Product
  Subsystem : Subsystem
  Switch{9..11,13} (4 alike) : Switch  Criteria=u2 ~= 0
  iLFault Switch : MultiPortSwitch  DataPortOrder=Zero-based contiguous  DataPortForDefault=Additional data port  zeroidx=on
  output : Outport
  wires:
  input/1 -> Product/1, Switch11/3, Switch10/3, iLFault Switch/2, iLFault Switch/5
  Constant9/1 -> Switch10/1
  Switch13/1 -> Switch9/2
  Switch9/1 -> output/1
  Switch11/1 -> iLFault Switch/4
  Constant11/1 -> Switch13/3
  iLFault Switch/1 -> Switch9/3, Subsystem/1(input)
  Switch10/1 -> iLFault Switch/3
  FaultStep/1 -> Switch10/2, Switch11/2
  NoiseStep/1 -> Switch13/1
  FaultSwtich/1 -> iLFault Switch/1
  NoiseFaultSwitch/1 -> Switch13/2
  Product/1 -> Switch11/1
  FaultFactor/1 -> Product/2
  Subsystem/1(noiseOutput) -> Switch9/1
